simulink model "simulation_case"  (R2019b)
settings: Solver=ode4  StartTime=0.0  StopTime=200  FixedStep=0.1  RelTol=1e-3
values from neighbouring files (symbols this model uses):
  A = [0,       1 ... (first row only)    [linear_system.m]    (also in system_used_for_case.m = [0,1)
  B = [0;omega^2]*gain    [linear_system.m]    (also in system_used_for_case.m = [0;omega_n^2]*gain)
  C = [1, 0]    [controller.m]    (also in linear_system.m; system_used_for_case.m = [1,0])
  Kd = K_lqr(1:end-1)    [system_used_for_case.m]
  Ki = -K_lqr(end)    [system_used_for_case.m]
  Ts = 1    [system_used_for_case.m]
settings Model: Creator=45427  LastModifiedBy=45427

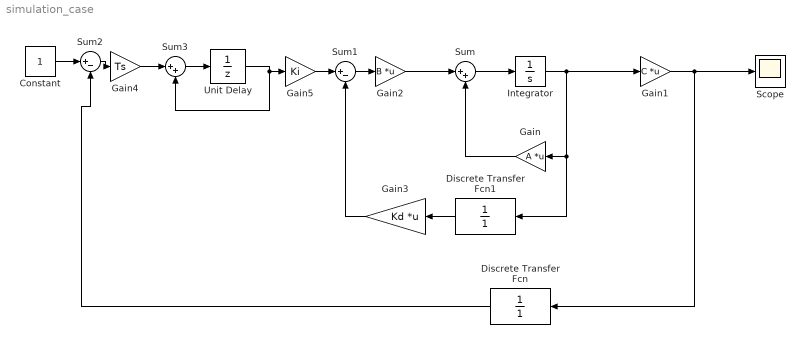
== system simulation_case ==
  Constant : Constant
  Discrete Transfer Fcn : DiscreteTransferFcn  Denominator=[1]  SampleTime=Ts
  Discrete Transfer Fcn1 : DiscreteTransferFcn  Denominator=[1]  SampleTime=Ts
  Gain : Gain  Gain=A  Multiplication=Matrix(K*u) (u vector)
  Gain1 : Gain  Gain=C  Multiplication=Matrix(K*u) (u vector)
  Gain2 : Gain  Gain=B  Multiplication=Matrix(K*u) (u vector)
  Gain3 : Gain  Gain=Kd  Multiplication=Matrix(K*u) (u vector)
  Gain4 : Gain  Gain=Ts
  Gain5 : Gain  Gain=Ki
  Integrator : Integrator
  Scope : Scope
  Sum : Sum  Inputs=|++
  Sum1 : Sum  Inputs=|+-
  Sum2 : Sum  Inputs=|+-
  Sum3 : Sum  Inputs=|++
  Unit Delay : UnitDelay  SampleTime=Ts  HasFrameUpgradeWarning=on
  wires:
  Sum/1 -> Integrator/1
  Gain/1 -> Sum/2
  Integrator/1 -> Discrete Transfer Fcn1/1, Gain/1, Gain1/1
  Gain2/1 -> Sum/1
  Sum1/1 -> Gain2/1
  Gain3/1 -> Sum1/2
  Constant/1 -> Sum2/1
  Gain1/1 -> Scope/1, Discrete Transfer Fcn/1
  Sum2/1 -> Gain4/1
  Gain4/1 -> Sum3/1
  Sum3/1 -> Unit Delay/1
  Unit Delay/1 -> Gain5/1, Sum3/2
  Gain5/1 -> Sum1/1
  Discrete Transfer Fcn/1 -> Sum2/2
  Discrete Transfer Fcn1/1 -> Gain3/1
